simulink model "on_off"  (R2017a)
settings: Solver=FixedStepAuto  StartTime=0.0  StopTime=50  FixedStep=0.01  RelTol=1e-3
undefined symbols (not defined in the file): C, R, ref
settings Model: Creator=Fikret Şafak  LastModifiedBy=baros

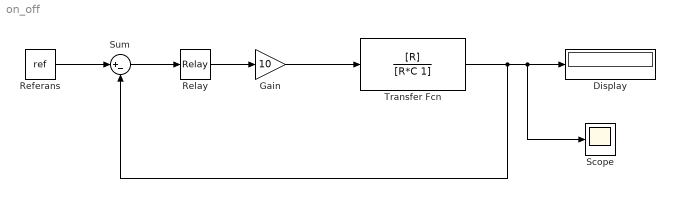
== system on_off ==
  Display : Display
  Gain : Gain  Gain=10
  Referans : Constant  Value=ref
  Relay : Relay  OnSwitchValue=0.5  OffSwitchValue=-0.5
  Scope : Scope
  Sum : Sum  Inputs=|+-
  Transfer Fcn : TransferFcn  Numerator=[R]  Denominator=[R*C 1]
  wires:
  Referans/1 -> Sum/1
  Sum/1 -> Relay/1
  Gain/1 -> Transfer Fcn/1
  Transfer Fcn/1 -> Scope/1, Display/1, Sum/2
  Relay/1 -> Gain/1
